simulink model "uav_simulation_tarot"  (R2020a)
settings: Solver=VariableStepAuto  StartTime=0.0  StopTime=sim_params.max_sim_time  FixedStep=uav.dynamics_srate  MaxStep=uav.dynamics_srate  MinStep=.01  RelTol=1e-3
undefined symbols (not defined in the file): deg, DiscIntNeverNeededParam, processes, rad, s, sim_params, trajectory, uav
libraries: aerolibconvert2 x2, shared6dof x1
(part 2 of 2)

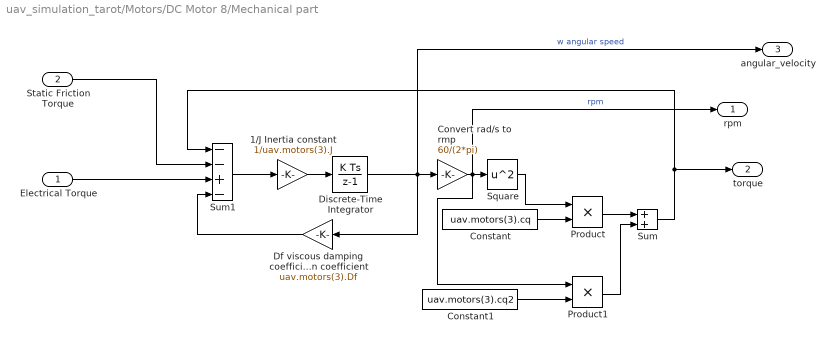
== system uav_simulation_tarot/Motors/DC Motor 8/Mechanical part ==
  Electrical Torque : Inport
  Static Friction Torque : Inport  Port=2
  1/J Inertia constant : Gain  Gain=1/uav.motors(3).J
  Constant : Constant  Value=uav.motors(3).cq
  Constant1 : Constant  Value=uav.motors(3).cq2
  Convert rad/s to rmp : Gain  Gain=60/(2*pi)
  "Df viscous damping coefficient Dynamic Friction coefficient " : Gain  Gain=uav.motors(3).Df
  Discrete-Time Integrator : DiscreteIntegrator  gainval=1  InitialCondition=sim_params.initial_conditions.w3  SampleTime=uav.dynamics_srate  ICPrevOutput=DiscIntNeverNeededParam  ICPrevScaledInput=DiscIntNeverNeededParam
  Product : Product
  Product1 : Product
  Square : Math  Operator=square  SaturateOnIntegerOverflow=on
  Sum : Sum
  Sum1 : Sum  Inputs=--+-
  rpm : Outport  VectorParamsAs1DForOutWhenUnconnected=off
  torque : Outport  Port=2
  angular_velocity : Outport  Port=3
  wires:
  1/J Inertia constant/1 -> Discrete-Time Integrator/1
  Static Friction Torque/1 -> Sum1/2
  "Df viscous damping coefficient Dynamic Friction coefficient "/1 -> Sum1/4
  Discrete-Time Integrator/1 -> angular_velocity/1, Convert rad/s to rmp/1, "Df viscous damping coefficient Dynamic Friction coefficient "/1  "w angular speed"
  Sum1/1 -> 1/J Inertia constant/1
  Electrical Torque/1 -> Sum1/3
  Sum/1 -> torque/1, Sum1/1
  Square/1 -> Product/1
  Constant/1 -> Product/2
  Product/1 -> Sum/1
  Constant1/1 -> Product1/2
  Convert rad/s to rmp/1 -> rpm/1, Product1/1, Square/1  "rpm"
  Product1/1 -> Sum/2

== matlab function uav_simulation_tarot/Subsystem/MATLAB Function1 ==
  settings: updateMethod=DISCRETE  sampleTime=.2
  data: mu input; y output; sigma input
function y = addNoise(mu, sigma)

y = normrnd(mu, sigma);

== matlab function uav_simulation_tarot/Forces and Moments Calculation ==
  data: w1 input; Fx output; w2 input; w3 input; w4 input; w5 input; w6 input; Fy output; Fz output; Mx output; My output; Mz output; w7 input; w8 input; Phi input; The input; Psi input
function [Fx,Fy,Fz,Mx,My,Mz] = fcn(w1,w2,w3,w4,w5,w6,w7,w8,Phi,The,Psi)
octomodel.g=9.80;
octomodel.m_t=10.66;
octomodel.l=0.635;
% Phi,The,Psi, in rad
w  = [w1; w2; w3; w4;w5; w6; w7; w8];

%% not used
%to fix numerical issues
%w=round(w,2);
% transform rpm to rad/s
%w=w./(60/(2*pi));

%% thrust generated by rotors

% Approach 1
% coef_t = 0.065;
%thrust = coef_t * density of air * velocity^2 * propeller diameter (m) ^4
%velocity in rev/sec, where  1 rev/sec = 1 rpm/60
%T = coef_t*1.225*((w./60).^2)*.47^4; % 18.5 inches ~ 0.47 m

% Approach 2
% thrust motor constant [Ns^2/rad^2]
b=9.8419e-05; % 
T = b.*((2*pi).*w./60).^2;

% total thrust generated by rotors
T_total=sum(T);
T_total=round(T_total*100)/100;

%% Forces in the local frame 
R_b_e = [cos(Psi)*cos(The) cos(Psi)*sin(The)*sin(Phi)-sin(Psi)*cos(Phi) cos(Psi)*sin(The)*cos(Phi)+sin(Psi)*sin(Phi);
       sin(Psi)*cos(The) sin(Psi)*sin(The)*sin(Phi)+cos(Psi)*cos(Phi) sin(Psi)*sin(The)*cos(Phi)-cos(Psi)*sin(Phi);
       -sin(The)         cos(The)*sin(Phi)                            cos(The)*cos(Phi)]; % Rib

Ftot_b=R_b_e'*[0 ;0; -octomodel.m_t*octomodel.g]+[0; 0; T_total]; 
Fx=Ftot_b(1);Fy=Ftot_b(2);Fz=Ftot_b(3);

%% Moments in the local frame 
% moment of each rotor
% Approach 1
%M = (2.138e-08)*w.^2 + (-1.279e-05)*w ;

% Approach 2
% rotor drag constant [Nms^2/rad^2]
d=1.8503e-06; % 
M = d.*((2*pi).*w./60).^2;


% torque generated by rotors
%motor angles
angsm=cos(pi/8); % 22.5 
anglg=cos(3*pi/8); % 67.5

Mx=octomodel.l*(T(1)*anglg +T(2)*angsm -T(3)*angsm -T(4)*anglg -T(5)*anglg ...
    -T(6)*angsm +T(7)*angsm +T(8)*anglg);%Tau_roll

My=octomodel.l*(-T(1)*angsm -T(2)*anglg -T(3)*anglg -T(4)*angsm +T(5)*angsm ...
    +T(6)*anglg +T(7)*anglg +T(8)*angsm);%Tau_theta

Mz= M(1) -M(2) +M(3) -M(4) +M(5) -M(6) +M(7) -M(8);%%Tau_yaw
end

== matlab function uav_simulation_tarot/arrival condition ==
  data: currentpos input; arrived output; dest input
function arrived = fcn(currentpos,dest)

result=norm(currentpos-dest);
if result<1 % less than one meter from the goal
    arrived=1;
else
    arrived=0;
end

== matlab function uav_simulation_tarot/Control allocation ==
  data: Fx input; wref1 output; Fy input; Fz input; Troll input; Tpitch input; Tyaw input; wref2 output; wref3 output; wref4 output; wref5 output; wref6 output; wref7 output; wref8 output
function [wref1,wref2,wref3,wref4,wref5,wref6,wref7,wref8] = fcn(Fx,Fy,Fz,Troll,Tpitch,Tyaw)
%% parameters 
%Maximum speed that the motors can reach in rad/s
Max_speed=670;

% arm length - distances from the octorotor center of mass ...
%        to the center of mass of all its rotors are equal and denoted by l.
l=0.635;
% thrust motor constant [Ns^2/rad^2]
b=9.8419e-05; % 
% rotor drag constant [Nms^2/rad^2]
d=1.8503e-06; % 

%angles
angsm=cos(pi/8); % 22.5 
anglg=cos(3*pi/8); % 67.5

% control allocation matrix
A_f=[b b b b b b b b; ...
    b*l*anglg b*l*angsm -b*l*angsm -b*l*anglg -b*l*anglg -b*l*angsm b*l*angsm b*l*anglg; ...
    -b*l*angsm -b*l*anglg -b*l*anglg -b*l*angsm b*l*angsm b*l*anglg b*l*anglg b*l*angsm; ...
    d -d d -d d -d d -d];

%desired input
u_des=[Fz;Troll;Tpitch;Tyaw];

%control allocation
Omega_s=pinv(A_f)*u_des; %inverse of A_f is A_f\

% velocity checking
wref=zeros(8);
for i=1:length(Omega_s)
    if Omega_s(i)<0
        wref(i)=0;
    elseif Omega_s(i)>Max_speed^2
        wref(i)=Max_speed;
    else
        wref(i)=sqrt(Omega_s(i));
    end
end

%velocity assignment in V
% multiply=0.0384615; 
multiply=0.0325;
for i=1:length(wref)
    % voltage saturation check
    if(wref(i)*multiply > 26.1)
        wref(i)=26.1;
    else
        wref(i)=wref(i)*multiply;
    end
end

wref1=wref(1);
wref2=wref(2);
wref3=wref(3);
wref4=wref(4);
wref5=wref(5);
wref6=wref(6);
wref7=wref(7);
wref8=wref(8);







% %% parameters required
% % load('params/octoModel.mat');
% gamma=3;%octomodel.tiltmotorangle;
% alpha=45;%octomodel.separationmotorangle;
% dl=0.45;%octomodel.dl;
% constant=(1/sqrt(2));
% ds=0.35;%octomodel.ds;
% ct=3.4262e-05;%octomodel.ct*(60/(2*pi))^2 -> in octomodel is for rpm, here I need it in rad/s;
% cq=9.3846e-07;%octomodel.cq*(60/(2*pi))^2 -> in octomodel is for rpm, here I need it in rad/s;
% 
% %% rotation matrices because of 3 degrees tilted angle
% 
% E_m_b = [0 -sin(alpha)*sin(gamma) sin(gamma) -cos(alpha)*sin(gamma) 0 sin(alpha)*sin(gamma) -sin(gamma) cos(alpha)*sin(gamma);
%          -sin(gamma)  cos(alpha)*sin(gamma) 0 -sin(alpha)*sin(gamma) sin(gamma) -cos(alpha)*sin(gamma) 0 sin(alpha)*sin(gamma);
%          -cos(gamma) -cos(gamma) -cos(gamma) -cos(gamma) -cos(gamma) -cos(gamma) -cos(gamma) -cos(gamma)];
% 
% R_m=[dl 0 0; ...
%     constant*ds constant*ds 0; ...
%     0 dl 0; ...
%     -constant*ds constant*ds 0; ...
%     -dl 0 0; ...
%     -constant*ds -constant*ds 0; ...
%     0 -dl 0; ...
%     constant*ds -constant*ds 0]';
% 
% %% first form delta_b matrix
% %a vectors
% a=zeros(3,8);
% for i=1:8
%     e_i_b=E_m_b(:,i);
%     a(:,i)=(ct).*e_i_b;
% end
% 
% %b vectors
% b=zeros(3,8);
% for i=1:8
%     e_i_b=E_m_b(:,i);
%     r_m=R_m(:,i);
%     b(:,i)=cross( r_m,(ct).*e_i_b ) + ((-1)^(i+1)*(cq)).*e_i_b;    
% end
% 
% %form matrix
% delta_b=[a;b];
% 
% %find pseudo-inverse
% delta_binv = pinv(delta_b);
% 
% %% calculate required w_ref
% Forces=[Fx,Fy,Fz];
% Torques=[Troll,Tpitch,Tyaw];
% if Troll>0
%     see=1;
% end
% input=[Forces,Torques]';
% wref=delta_binv*input;
% %check if complex
% if(isreal(wref(2)))
%     see=1;
% end
% 
% if length(find(wref<0))>0
%     pos=find(wref<0);
%     wref(pos)=0;
% end
% wref=sqrt(wref);
% 
% % %angular velocity in rad/s
% % wref1=wref(1);
% % wref2=wref(2);
% % wref3=wref(3);
% % wref4=wref(4);
% % wref5=wref(5);
% % wref6=wref(6);
% % wref7=wref(7);
% % wref8=wref(8);
% 
% %angular velocity in rpm
% % wref1=wref(1)*(60/(2*pi));
% % wref2=wref(2)*(60/(2*pi));
% % wref3=wref(3)*(60/(2*pi));
% % wref4=wref(4)*(60/(2*pi));
% % wref5=wref(5)*(60/(2*pi));
% % wref6=wref(6)*(60/(2*pi));
% % wref7=wref(7)*(60/(2*pi));
% % wref8=wref(8)*(60/(2*pi));
% 
% %% now convert to voltage in the range 0-22V
% % divide=36.17; %true is 36.37
% % multiply=0.0238; %for 8800 rpm nominal 
% multiply=0.02762; %for 6783 rpm considering torque load 
% wref1=wref(1)*multiply;
% wref2=wref(2)*multiply;
% wref3=wref(3)*multiply;
% wref4=wref(4)*multiply;
% wref5=wref(5)*multiply;
% wref6=wref(6)*multiply;
% wref7=wref(7)*multiply;
% wref8=wref(8)*multiply;
% 
% see=1;

end

== matlab function uav_simulation_tarot/Adding noise ==
  data: u input; y output; t input
function y = fcn(u,t)
if t==2.99
    see=1;
end
y = zeros(6,1);
% posnoisestd=0.75; % gives maximum and minimum of +-3 meters
posnoisestd=0.1; % gives maximum and minimum of +-.5 meters
velnoisestd=0.005;
noisepos=posnoisestd.*randn(3,1);
noisevel=velnoisestd.*randn(3,1);
noise=[noisepos ;noisevel];
y = y + u + noise;
